simulink model "BloquesParkDirecta"  (R2023b)
settings: Solver=VariableStepAuto  StartTime=0.0  StopTime=10.0  RelTol=1e-3
values from neighbouring files (symbols this model uses):
  P_p = 3    [Parametros.m]
settings Model: Creator=Home  LastModifiedBy=Home

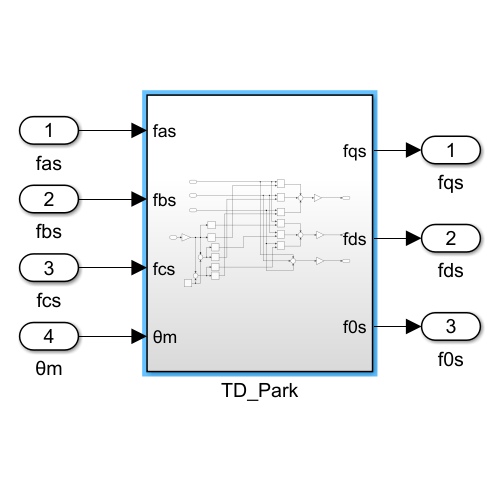
[thumbnail: Simulink's stored preview of the top-level diagram]
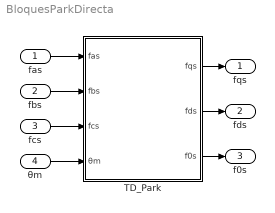
== system BloquesParkDirecta ==
  fas : Inport
  fbs : Inport  Port=2
  fcs : Inport  Port=3
  θm : Inport  Port=4
  TD_Park : Subsystem
  fqs : Outport
  fds : Outport  Port=2
  f0s : Outport  Port=3
  wires:
  fas/1 -> TD_Park/1(fas)
  fbs/1 -> TD_Park/2(fbs)
  fcs/1 -> TD_Park/3(fcs)
  θm/1 -> TD_Park/4(θm)
  TD_Park/1(fqs) -> fqs/1
  TD_Park/2(fds) -> fds/1
  TD_Park/3(f0s) -> f0s/1

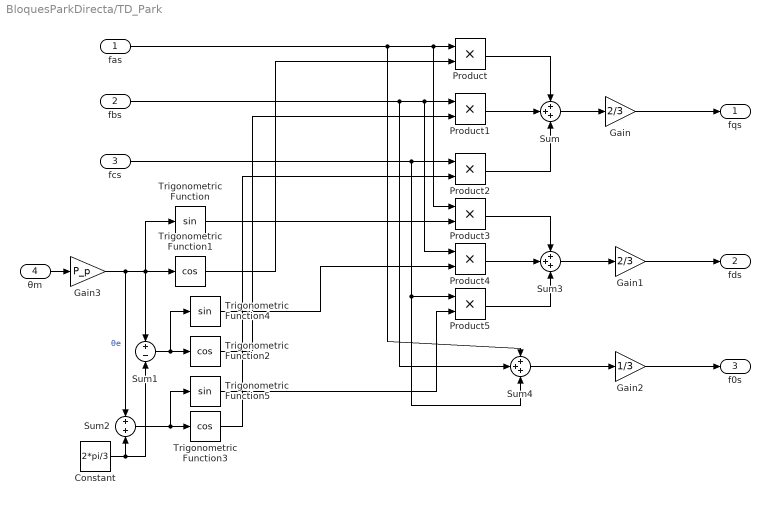
== system BloquesParkDirecta/TD_Park ==
  fas : Inport
  fbs : Inport  Port=2
  fcs : Inport  Port=3
  θm : Inport  Port=4
  Constant : Constant  Value=2*pi/3
  Gain : Gain  Gain=2/3
  Gain1 : Gain  Gain=2/3
  Gain2 : Gain  Gain=1/3
  Gain3 : Gain  Gain=P_p
  Product{,1..5} (6 alike) : Product
  Sum : Sum  Inputs=+++
  Sum1 : Sum  Inputs=+-
  Sum2 : Sum
  Sum3 : Sum  Inputs=+++
  Sum4 : Sum  Inputs=+++
  Trigonometric Function : Trigonometry
  Trigonometric Function1 : Trigonometry  Operator=cos
  Trigonometric Function2 : Trigonometry  Operator=cos
  Trigonometric Function3 : Trigonometry  Operator=cos
  Trigonometric Function4 : Trigonometry
  Trigonometric Function5 : Trigonometry
  fqs : Outport
  fds : Outport  Port=2
  f0s : Outport  Port=3
  wires:
  fas/1 -> Sum4/1, Product3/1, Product/1
  Trigonometric Function3/1 -> Product2/2
  Sum1/1 -> Trigonometric Function4/1, Trigonometric Function2/1
  Constant/1 -> Sum2/2, Sum1/2
  Trigonometric Function1/1 -> Product/2
  fcs/1 -> Product5/1, Sum4/3, Product2/1
  θm/1 -> Gain3/1
  Product5/1 -> Sum3/3
  Product/1 -> Sum/1
  Product3/1 -> Sum3/1
  Product1/1 -> Sum/2
  Trigonometric Function/1 -> Product3/2
  Sum2/1 -> Trigonometric Function5/1, Trigonometric Function3/1
  Trigonometric Function5/1 -> Product5/2
  Sum4/1 -> Gain2/1
  fbs/1 -> Sum4/2, Product4/1, Product1/1
  Product2/1 -> Sum/3
  Gain/1 -> fqs/1
  Trigonometric Function4/1 -> Product4/2
  Product4/1 -> Sum3/2
  Trigonometric Function2/1 -> Product1/2
  Gain2/1 -> f0s/1
  Sum/1 -> Gain/1
  Gain1/1 -> fds/1
  Sum3/1 -> Gain1/1
  Gain3/1 -> Sum2/1, Trigonometric Function/1, Sum1/1, Trigonometric Function1/1  "θe"
